simulink model "GB_and_guyan"  (R2023a)
settings: Solver=ode4  StartTime=0.0  StopTime=tend  FixedStep=dt  RelTol=1e-3
undefined symbols (not defined in the file): a0, a1, a2, a3, a4, a5, a6, a7, Ag, AgN, alpha1, alpha2, C_phys_5dof, CNrt, CRrt, delay, dt, dv1, dv2, EQ_intensity, EQ_sw, F, FN, K_phys_5dof, Kbar_inv, KNbar_inv, Koo, Kot, l, lN, M_phys_5dof, MNrt, MRrt, Muu, Phi_u, Rbar, RNbar
libraries: simulink x1, sldrtlib x1
settings Model: Creator=icu327  LastModifiedBy=liangyu
settings SolverCC: AlgebraicLoopSolver=TrustRegion
settings DataIOCC: SaveFormat=Array  ReturnWorkspaceOutputs=off
settings DebuggingCC: UnconnectedInputMsg=warning  UnconnectedOutputMsg=warning  UnconnectedLineMsg=warning  ArithmeticOperatorsInVariantConditions=warning
settings HardwareCC: ProdBitPerLong=64  ProdHWDeviceType=Intel->x86-64 (Linux 64)
settings ModelReferenceCC: EnableRefExpFcnMdlSchedulingChecks=on
settings SFSimCC: CustomCodeUndefinedFunction=UseInterfaceOnly
settings RTWCC: Description=Simulink Desktop Real-Time  SystemTargetFile=sldrt.tlc  TemplateMakefile=sldrt.tmf  RTWCompilerOptimization=on
settings CodeAppCC: MaxIdLength=95  StateflowObjectComments=on
settings SimulinkDesktopRealTimeCC: TargetLibSuffix=_sldrt.a  TargetPreCompLibLocation=C:\Program Files\MATLAB\R2023a\toolbox\sldrt\lib\win64

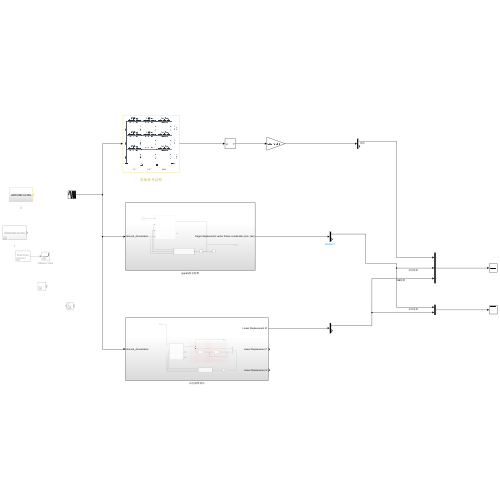
[thumbnail: Simulink's stored preview of the top-level diagram]
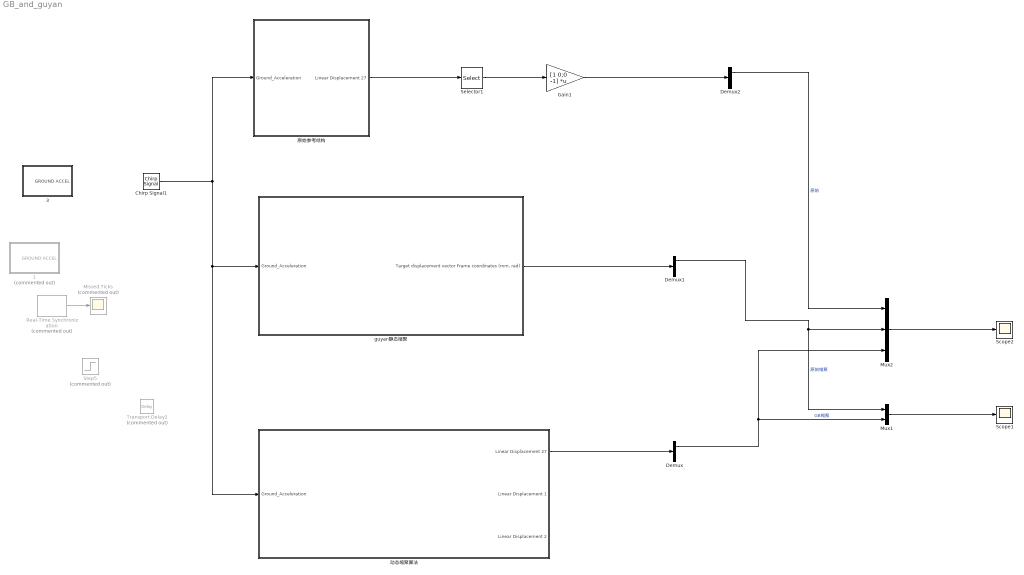
== system GB_and_guyan ==
  " 1" : Subsystem  Commented=on
  " 3" : Subsystem
  " 原始参考结构" : Subsystem
      mask Display: image('$imagefile'); % Use "Edit Image" on toolstrip to change.
  Chirp Signal1 : simulink/Sources/Chirp Signal  f1=0.1  T=60  f2=25
  Demux : Demux  Outputs=2
  Demux1 : Demux  Outputs=2
  Demux2 : Demux  Outputs=2
  Gain1 : Gain  Gain=[1 0;0 -1]  Multiplication=Matrix(K*u) (u vector)
  Missed Ticks : Scope  Commented=on
  Mux1 : Mux  Inputs=2
  Mux2 : Mux  Inputs=3
  Real-Time Synchronization : sldrtlib/Real-Time Synchronization  Commented=on  SampleTime=dt  MaxMissedTicks=10000  ShowMissedTicks=on  YieldWhenWaiting=off
  Scope1 : Scope
  Scope2 : Scope
  Selector1 : Selector  InputPortWidth=29  IndexOptions=Index vector (dialog)  Indices=[27 21]  OutputSizes=1
  Step5 : Step  Commented=on  SampleTime=0
  Transport Delay2 : TransportDelay  Commented=on  DelayTime=0.03
  guyan静态缩聚 : Subsystem
  动态缩聚算法 : Subsystem
  wires:
  Real-Time Synchronization/1 -> Missed Ticks/1
  " 原始参考结构"/1(Linear Displacement 27) -> Selector1/1
  Selector1/1 -> Gain1/1
  Chirp Signal1/1 -> 动态缩聚算法/1(Ground_Acceleration), guyan静态缩聚/1(Ground_Acceleration), " 原始参考结构"/1(Ground_Acceleration)
  Demux1/1 -> Mux2/2, Mux1/1  "原始缩聚"
  Mux1/1 -> Scope1/1
  Demux/1 -> Mux2/3, Mux1/2  "GB缩聚"
  Gain1/1 -> Demux2/1
  Demux2/1 -> Mux2/1  "原始"
  Mux2/1 -> Scope2/1
  guyan静态缩聚/1("Target displacement vector Frame coordinates (mm, rad)") -> Demux1/1
  动态缩聚算法/1(Linear Displacement 27) -> Demux/1

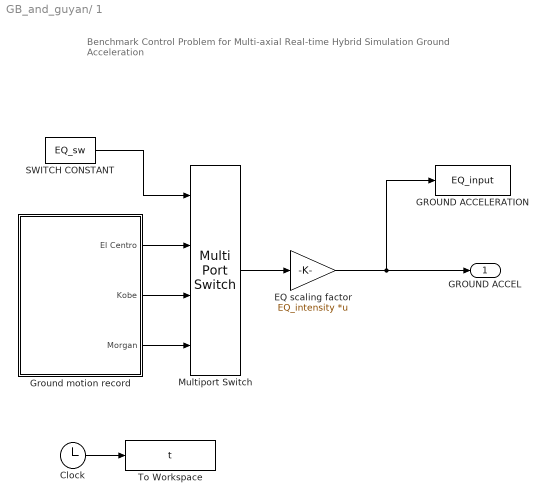
== system GB_and_guyan/ 1 ==
  note: Benchmark Control Problem for
      | Multi-axial Real-time Hybrid Simulation
      | Ground Acceleration
  Clock : Clock
  EQ scaling factor : Gain  Gain=EQ_intensity  Multiplication=Matrix(K*u)
  GROUND ACCELERATION : ToWorkspace  VariableName=EQ_input  SampleTime=-1
      settings: Save2DSignal=2-D array (concatenate along first dimension)
  Ground motion record : Subsystem
  Multiport Switch : MultiPortSwitch  SaturateOnIntegerOverflow=off  InputSameDT=off
  SWITCH CONSTANT : Constant  Value=EQ_sw
  To Workspace : ToWorkspace  VariableName=t  SampleTime=dt
  GROUND ACCEL : Outport  VectorParamsAs1DForOutWhenUnconnected=off
  wires:
  Multiport Switch/1 -> EQ scaling factor/1
  EQ scaling factor/1 -> GROUND ACCELERATION/1, GROUND ACCEL/1
  Ground motion record/1(El Centro) -> Multiport Switch/2
  Ground motion record/2(Kobe) -> Multiport Switch/3
  Ground motion record/3(Morgan) -> Multiport Switch/4
  SWITCH CONSTANT/1 -> Multiport Switch/1
  Clock/1 -> To Workspace/1

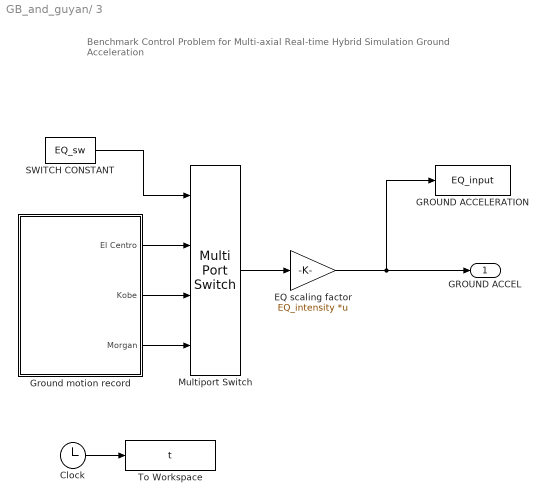
== system GB_and_guyan/ 3 ==
  note: Benchmark Control Problem for
      | Multi-axial Real-time Hybrid Simulation
      | Ground Acceleration
  Clock : Clock
  EQ scaling factor : Gain  Gain=EQ_intensity  Multiplication=Matrix(K*u)
  GROUND ACCELERATION : ToWorkspace  VariableName=EQ_input  SampleTime=-1
      settings: Save2DSignal=2-D array (concatenate along first dimension)
  Ground motion record : Subsystem
  Multiport Switch : MultiPortSwitch  SaturateOnIntegerOverflow=off  InputSameDT=off
  SWITCH CONSTANT : Constant  Value=EQ_sw
  To Workspace : ToWorkspace  VariableName=t  SampleTime=dt
  GROUND ACCEL : Outport  VectorParamsAs1DForOutWhenUnconnected=off
  wires:
  Multiport Switch/1 -> EQ scaling factor/1
  EQ scaling factor/1 -> GROUND ACCELERATION/1, GROUND ACCEL/1
  Ground motion record/1(El Centro) -> Multiport Switch/2
  Ground motion record/2(Kobe) -> Multiport Switch/3
  Ground motion record/3(Morgan) -> Multiport Switch/4
  SWITCH CONSTANT/1 -> Multiport Switch/1
  Clock/1 -> To Workspace/1

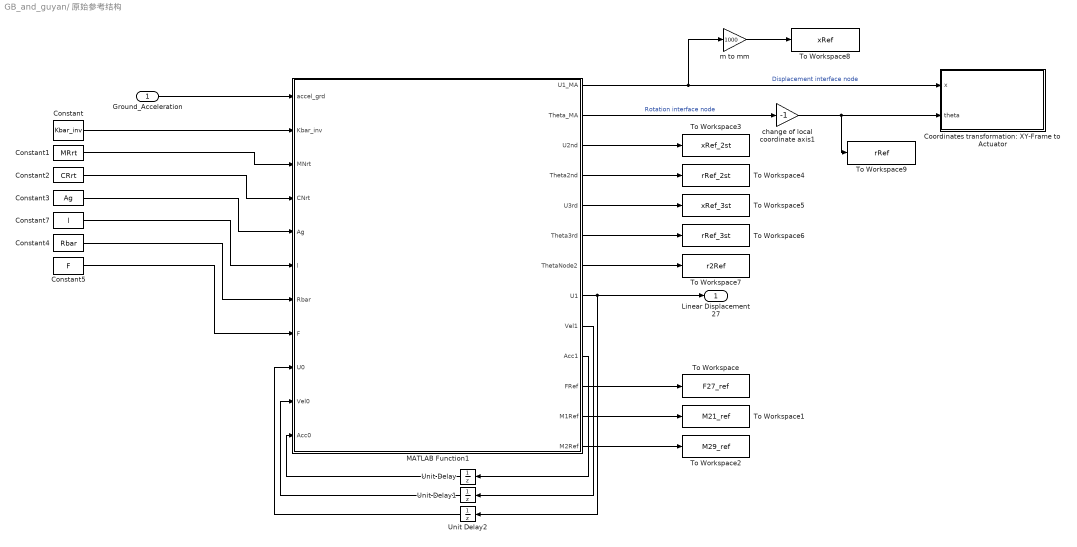
== system GB_and_guyan/ 原始参考结构 ==
  Ground_Acceleration : Inport
  Constant : Constant  Value=Kbar_inv  VectorParams1D=off
  Constant1 : Constant  Value=MRrt  VectorParams1D=off
  Constant2 : Constant  Value=CRrt  VectorParams1D=off
  Constant3 : Constant  Value=Ag  VectorParams1D=off
  Constant4 : Constant  Value=Rbar  VectorParams1D=off
  Constant5 : Constant  Value=F  VectorParams1D=off
  Constant7 : Constant  Value=l  VectorParams1D=off
  "Coordinates transformation: XY-Frame to Actuator " : Subsystem
  MATLAB Function1 : MATLAB Function  TreatAsAtomicUnit=on
  To Workspace : ToWorkspace  VariableName=F27_ref  SampleTime=-1
  To Workspace1 : ToWorkspace  VariableName=M21_ref  SampleTime=-1
  To Workspace2 : ToWorkspace  VariableName=M29_ref  SampleTime=-1
  To Workspace3 : ToWorkspace  VariableName=xRef_2st  SampleTime=dt
  To Workspace4 : ToWorkspace  VariableName=rRef_2st  SampleTime=dt
  To Workspace5 : ToWorkspace  VariableName=xRef_3st  SampleTime=dt
  To Workspace6 : ToWorkspace  VariableName=rRef_3st  SampleTime=dt
  To Workspace7 : ToWorkspace  VariableName=r2Ref  SampleTime=dt
  To Workspace8 : ToWorkspace  VariableName=xRef  SampleTime=dt
  To Workspace9 : ToWorkspace  VariableName=rRef  SampleTime=dt
  Unit Delay : UnitDelay  SampleTime=-1  HasFrameUpgradeWarning=on
  Unit Delay1 : UnitDelay  SampleTime=-1  HasFrameUpgradeWarning=on
  Unit Delay2 : UnitDelay  SampleTime=-1  HasFrameUpgradeWarning=on
  change of local coordinate axis1 : Gain  Gain=-1
  "m to mm  " : Gain  Gain=1000
  Linear Displacement 27 : Outport  VectorParamsAs1DForOutWhenUnconnected=off
  wires:
  Ground_Acceleration/1 -> MATLAB Function1/1(accel_grd)
  MATLAB Function1/1(U1_MA) -> "Coordinates transformation: XY-Frame to Actuator "/1(x), "m to mm  "/1  "Displacement interface node"
  MATLAB Function1/2(Theta_MA) -> change of local coordinate axis1/1  "Rotation interface node"
  Constant/1 -> MATLAB Function1/2(Kbar_inv)
  Constant1/1 -> MATLAB Function1/3(MNrt)
  Constant2/1 -> MATLAB Function1/4(CNrt)
  Constant3/1 -> MATLAB Function1/5(Ag)
  Constant7/1 -> MATLAB Function1/6(l)
  Constant4/1 -> MATLAB Function1/7(Rbar)
  Unit Delay2/1 -> MATLAB Function1/9(U0)
  Unit Delay1/1 -> MATLAB Function1/10(Vel0)
  Unit Delay/1 -> MATLAB Function1/11(Acc0)
  MATLAB Function1/9(Vel1) -> Unit Delay1/1
  MATLAB Function1/10(Acc1) -> Unit Delay/1
  MATLAB Function1/8(U1) -> Linear Displacement 27/1, Unit Delay2/1
  Constant5/1 -> MATLAB Function1/8(F)
  MATLAB Function1/13(M2Ref) -> To Workspace2/1
  MATLAB Function1/12(M1Ref) -> To Workspace1/1
  MATLAB Function1/11(FRef) -> To Workspace/1
  MATLAB Function1/3(U2nd) -> To Workspace3/1
  MATLAB Function1/4(Theta2nd) -> To Workspace4/1
  MATLAB Function1/5(U3rd) -> To Workspace5/1
  MATLAB Function1/6(Theta3rd) -> To Workspace6/1
  MATLAB Function1/7(ThetaNode2) -> To Workspace7/1
  "m to mm  "/1 -> To Workspace8/1
  change of local coordinate axis1/1 -> To Workspace9/1, "Coordinates transformation: XY-Frame to Actuator "/2(theta)

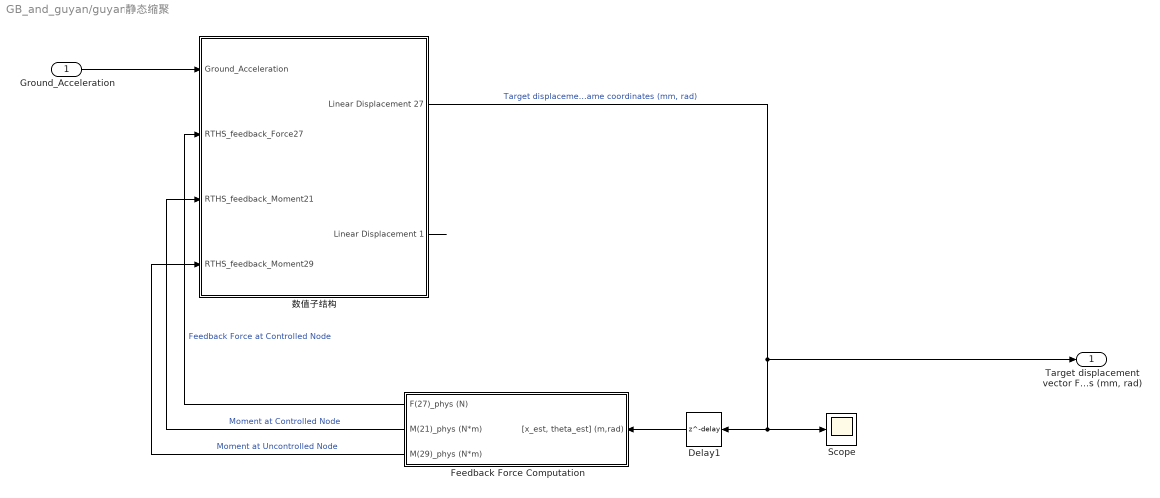
== system GB_and_guyan/guyan静态缩聚 ==
  Ground_Acceleration : Inport
  " 数值子结构" : Subsystem
      mask Display: image('$imagefile'); % Use "Edit Image" on toolstrip to change.
  Delay1 : Delay  DelayLength=delay
  Feedback Force Computation : Subsystem
  Scope : Scope
  "Target displacement vector Frame coordinates (mm, rad)" : Outport
  wires:
  Feedback Force Computation/2(M(21)_phys (N*m)) -> " 数值子结构"/3(RTHS_feedback_Moment21)  "Moment at Controlled Node"
  " 数值子结构"/1(Linear Displacement 27) -> "Target displacement vector Frame coordinates (mm, rad)"/1, Scope/1, Delay1/1  "Target displacement vector Frame coordinates (mm, rad)"
  Ground_Acceleration/1 -> " 数值子结构"/1(Ground_Acceleration)
  Feedback Force Computation/1(F(27)_phys (N)) -> " 数值子结构"/2(RTHS_feedback_Force27)  "Feedback Force at Controlled Node"
  Delay1/1 -> Feedback Force Computation/1("[x_est, theta_est] (m,rad)")
  Feedback Force Computation/3(M(29)_phys (N*m)) -> " 数值子结构"/4(RTHS_feedback_Moment29)  "Moment at Uncontrolled Node"
  " 数值子结构"/2(Linear Displacement 1) -> ?

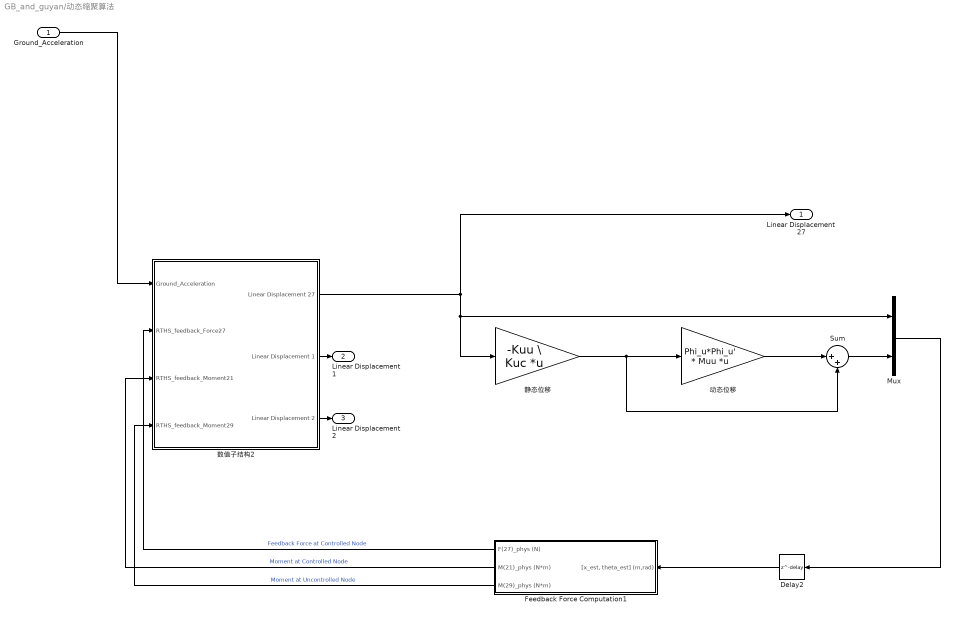
== system GB_and_guyan/动态缩聚算法 ==
  Ground_Acceleration : Inport
  " 数值子结构2" : Subsystem
      mask Display: image('$imagefile'); % Use "Edit Image" on toolstrip to change.
  Delay2 : Delay  DelayLength=delay
  Feedback Force Computation1 : Subsystem
  Mux : Mux  Inputs=2
  Sum : Sum  Inputs=|++
  动态位移 : Gain  Gain=Phi_u*Phi_u' * Muu  Multiplication=Matrix(K*u) (u vector)
  静态位移 : Gain  Gain=-Kuu \ Kuc  Multiplication=Matrix(K*u) (u vector)
  Linear Displacement 27 : Outport
  Linear Displacement 1 : Outport  Port=2
  Linear Displacement 2 : Outport  Port=3
  wires:
  动态位移/1 -> Sum/1
  " 数值子结构2"/1(Linear Displacement 27) -> Linear Displacement 27/1, 静态位移/1, Mux/1
  Feedback Force Computation1/3(M(29)_phys (N*m)) -> " 数值子结构2"/4(RTHS_feedback_Moment29)  "Moment at Uncontrolled Node"
  Mux/1 -> Delay2/1
  静态位移/1 -> 动态位移/1, Sum/2
  Sum/1 -> Mux/2
  Feedback Force Computation1/2(M(21)_phys (N*m)) -> " 数值子结构2"/3(RTHS_feedback_Moment21)  "Moment at Controlled Node"
  Delay2/1 -> Feedback Force Computation1/1("[x_est, theta_est] (m,rad)")
  Feedback Force Computation1/1(F(27)_phys (N)) -> " 数值子结构2"/2(RTHS_feedback_Force27)  "Feedback Force at Controlled Node"
  " 数值子结构2"/2(Linear Displacement 1) -> Linear Displacement 1/1
  " 数值子结构2"/3(Linear Displacement 2) -> Linear Displacement 2/1
  Ground_Acceleration/1 -> " 数值子结构2"/1(Ground_Acceleration)

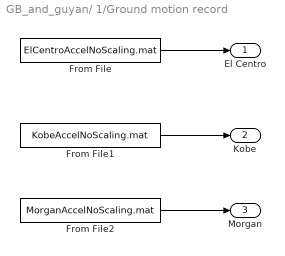
== system GB_and_guyan/ 1/Ground motion record ==
  From File : FromFile  FileName=ElCentroAccelNoScaling.mat  SampleTime=dt
  From File1 : FromFile  FileName=KobeAccelNoScaling.mat  SampleTime=dt
  From File2 : FromFile  FileName=MorganAccelNoScaling.mat  SampleTime=dt
  El Centro : Outport
  Kobe : Outport  Port=2
  Morgan : Outport  Port=3
  wires:
  From File/1 -> El Centro/1
  From File2/1 -> Morgan/1
  From File1/1 -> Kobe/1

== system GB_and_guyan/ 3/Ground motion record ==
  From File : FromFile  FileName=D:\matlab\LY\gitee\liangyustability\simulink模型修改\Ground_motions\ElCentroAccelNoScaling.mat  SampleTime=dt
  From File1 : FromFile  FileName=D:\matlab\LY\gitee\liangyustability\simulink模型修改\Ground_motions\KobeAccelNoScaling.mat  SampleTime=dt
  From File2 : FromFile  FileName=D:\matlab\LY\gitee\liangyustability\simulink模型修改\Ground_motions\MorganAccelNoScaling.mat  SampleTime=dt
  El Centro : Outport
  Kobe : Outport  Port=2
  Morgan : Outport  Port=3
  wires:
  From File/1 -> El Centro/1
  From File2/1 -> Morgan/1
  From File1/1 -> Kobe/1

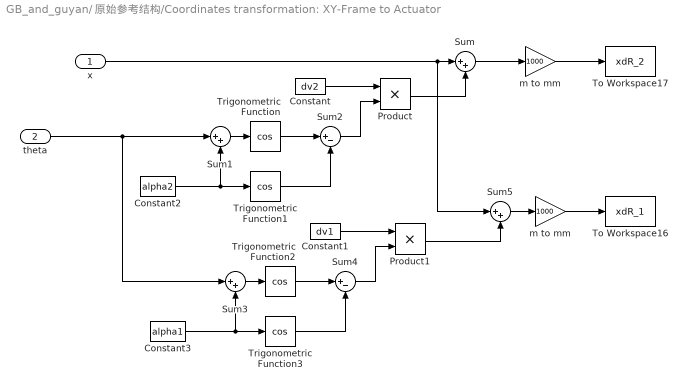
== system GB_and_guyan/ 原始参考结构/Coordinates transformation: XY-Frame to Actuator  ==
  x : Inport
  theta : Inport  Port=2
  Constant : Constant  Value=dv2
  Constant1 : Constant  Value=dv1
  Constant2 : Constant  Value=alpha2
  Constant3 : Constant  Value=alpha1
  Product : Product
  Product1 : Product
  Sum{,1,3,5} (4 alike) : Sum  Inputs=|++
  Sum2 : Sum  Inputs=|+-
  Sum4 : Sum  Inputs=|+-
  To Workspace16 : ToWorkspace  VariableName=xdR_1  SampleTime=dt
  To Workspace17 : ToWorkspace  VariableName=xdR_2  SampleTime=dt
  Trigonometric Function{,1..3} (4 alike) : Trigonometry  Operator=cos
  m to mm : Gain  Gain=1000
  "m to mm " : Gain  Gain=1000
  wires:
  theta/1 -> Sum1/1, Sum3/1
  "m to mm "/1 -> To Workspace16/1
  m to mm/1 -> To Workspace17/1
  Sum5/1 -> "m to mm "/1
  Product1/1 -> Sum5/2
  Constant1/1 -> Product1/1
  Constant3/1 -> Trigonometric Function3/1, Sum3/2
  Sum3/1 -> Trigonometric Function2/1
  Trigonometric Function2/1 -> Sum4/1
  Trigonometric Function3/1 -> Sum4/2
  Sum4/1 -> Product1/2
  Sum/1 -> m to mm/1
  Product/1 -> Sum/2
  Sum2/1 -> Product/2
  Trigonometric Function1/1 -> Sum2/2
  Trigonometric Function/1 -> Sum2/1
  Sum1/1 -> Trigonometric Function/1
  Constant2/1 -> Trigonometric Function1/1, Sum1/2
  Constant/1 -> Product/1
  x/1 -> Sum/1, Sum5/1

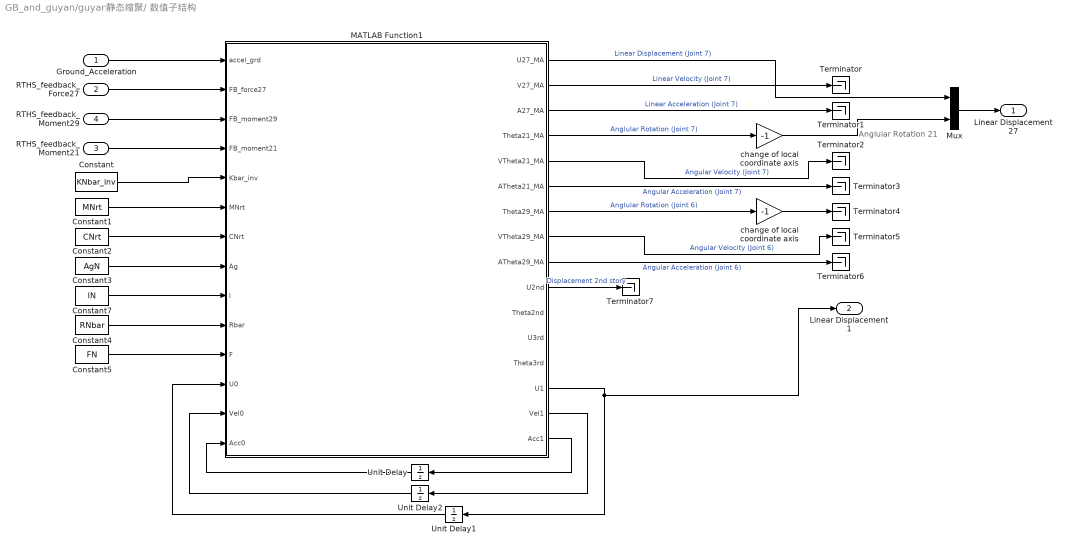
== system GB_and_guyan/guyan静态缩聚/ 数值子结构 ==
  note: Anglular Rotation 21
  Ground_Acceleration : Inport
  RTHS_feedback_Force27 : Inport  Port=2
  RTHS_feedback_Moment21 : Inport  Port=3
  RTHS_feedback_Moment29 : Inport  Port=4
  Constant : Constant  Value=KNbar_inv  VectorParams1D=off
  Constant1 : Constant  Value=MNrt  VectorParams1D=off
  Constant2 : Constant  Value=CNrt  VectorParams1D=off
  Constant3 : Constant  Value=AgN  VectorParams1D=off
  Constant4 : Constant  Value=RNbar  VectorParams1D=off
  Constant5 : Constant  Value=FN  VectorParams1D=off
  Constant7 : Constant  Value=lN  VectorParams1D=off
  MATLAB Function1 : MATLAB Function  TreatAsAtomicUnit=on
  Mux : Mux  Inputs=2
  Terminator{,1..7} (8 alike) : Terminator
  Unit Delay : UnitDelay  SampleTime=-1  HasFrameUpgradeWarning=on
  Unit Delay1 : UnitDelay  SampleTime=-1  HasFrameUpgradeWarning=on
  Unit Delay2 : UnitDelay  SampleTime=-1  HasFrameUpgradeWarning=on
  change of local coordinate axis : Gain  Gain=-1
  "change of local coordinate axis  " : Gain  Gain=-1
  Linear Displacement 27 : Outport  VectorParamsAs1DForOutWhenUnconnected=off
  Linear Displacement 1 : Outport  Port=2  VectorParamsAs1DForOutWhenUnconnected=off
  wires:
  Ground_Acceleration/1 -> MATLAB Function1/1(accel_grd)
  RTHS_feedback_Force27/1 -> MATLAB Function1/2(FB_force27)
  RTHS_feedback_Moment29/1 -> MATLAB Function1/3(FB_moment29)
  MATLAB Function1/1(U27_MA) -> Mux/1  "Linear Displacement (Joint 7)"
  MATLAB Function1/4(Theta21_MA) -> change of local coordinate axis/1  "Anglular Rotation (Joint 7)"
  Constant/1 -> MATLAB Function1/5(Kbar_inv)
  Constant1/1 -> MATLAB Function1/6(MNrt)
  Constant2/1 -> MATLAB Function1/7(CNrt)
  Constant3/1 -> MATLAB Function1/8(Ag)
  Constant7/1 -> MATLAB Function1/9(l)
  Constant4/1 -> MATLAB Function1/10(Rbar)
  Unit Delay1/1 -> MATLAB Function1/12(U0)
  Unit Delay2/1 -> MATLAB Function1/13(Vel0)
  Unit Delay/1 -> MATLAB Function1/14(Acc0)
  MATLAB Function1/15(Vel1) -> Unit Delay2/1
  MATLAB Function1/16(Acc1) -> Unit Delay/1
  Constant5/1 -> MATLAB Function1/11(F)
  MATLAB Function1/2(V27_MA) -> Terminator/1  "Linear Velocity (Joint 7)"
  MATLAB Function1/3(A27_MA) -> Terminator1/1  "Linear Acceleration (Joint 7)"
  MATLAB Function1/5(VTheta21_MA) -> Terminator2/1  "Angular Velocity (Joint 7)"
  MATLAB Function1/6(ATheta21_MA) -> Terminator3/1  "Angular Acceleration (Joint 7)"
  MATLAB Function1/9(ATheta29_MA) -> Terminator6/1  "Angular Acceleration (Joint 6)"
  MATLAB Function1/8(VTheta29_MA) -> Terminator5/1  "Angular Velocity (Joint 6)"
  MATLAB Function1/7(Theta29_MA) -> "change of local coordinate axis  "/1  "Anglular Rotation (Joint 6)"
  RTHS_feedback_Moment21/1 -> MATLAB Function1/4(FB_moment21)
  change of local coordinate axis/1 -> Mux/2
  "change of local coordinate axis  "/1 -> Terminator4/1
  Mux/1 -> Linear Displacement 27/1
  MATLAB Function1/10(U2nd) -> Terminator7/1  "Displacement 2nd story"
  MATLAB Function1/14(U1) -> Linear Displacement 1/1, Unit Delay1/1

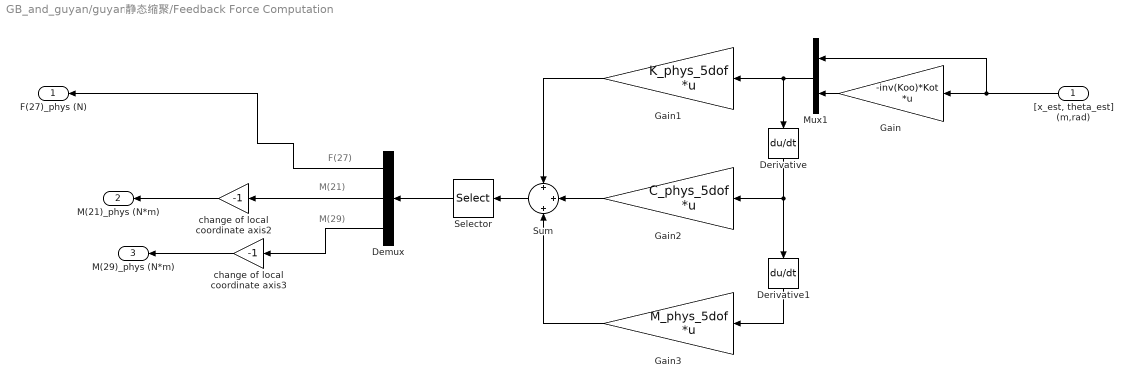
== system GB_and_guyan/guyan静态缩聚/Feedback Force Computation ==
  note: F(27)
  note: M(21)
  note: M(29)
  "[x_est, theta_est] (m,rad)" : Inport
  Demux : Demux  Outputs=3
  Derivative : Derivative
  Derivative1 : Derivative
  Gain : Gain  Gain=-inv(Koo)*Kot  Multiplication=Matrix(K*u) (u vector)
  Gain1 : Gain  Gain=K_phys_5dof  Multiplication=Matrix(K*u) (u vector)
  Gain2 : Gain  Gain=C_phys_5dof  Multiplication=Matrix(K*u) (u vector)
  Gain3 : Gain  Gain=M_phys_5dof  Multiplication=Matrix(K*u) (u vector)
  Mux1 : Mux  Inputs=2
  Selector : Selector  InputPortWidth=5  IndexOptions=Index vector (dialog)  Indices=[1 2 3]  OutputSizes=1
  Sum : Sum  Inputs=+|+|+
  change of local coordinate axis2 : Gain  Gain=-1
  change of local coordinate axis3 : Gain  Gain=-1
  F(27)_phys (N) : Outport  VectorParamsAs1DForOutWhenUnconnected=off
  M(21)_phys (N*m) : Outport  Port=2  VectorParamsAs1DForOutWhenUnconnected=off
  M(29)_phys (N*m) : Outport  Port=3  VectorParamsAs1DForOutWhenUnconnected=off
  wires:
  Gain/1 -> Mux1/2
  Derivative1/1 -> Gain3/1
  Gain2/1 -> Sum/2
  Derivative/1 -> Gain2/1, Derivative1/1
  Gain1/1 -> Sum/1
  "[x_est, theta_est] (m,rad)"/1 -> Gain/1, Mux1/1
  Demux/1 -> F(27)_phys (N)/1
  Sum/1 -> Selector/1
  Selector/1 -> Demux/1
  Gain3/1 -> Sum/3
  Demux/2 -> change of local coordinate axis2/1
  Demux/3 -> change of local coordinate axis3/1
  Mux1/1 -> Derivative/1, Gain1/1
  change of local coordinate axis2/1 -> M(21)_phys (N*m)/1
  change of local coordinate axis3/1 -> M(29)_phys (N*m)/1

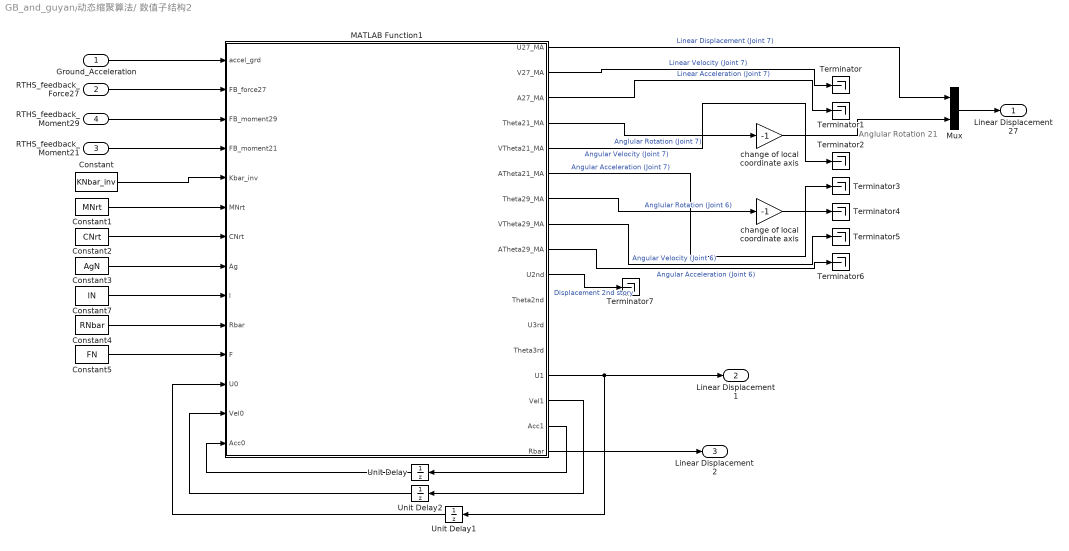
== system GB_and_guyan/动态缩聚算法/ 数值子结构2 ==
  note: Anglular Rotation 21
  Ground_Acceleration : Inport
  RTHS_feedback_Force27 : Inport  Port=2
  RTHS_feedback_Moment21 : Inport  Port=3
  RTHS_feedback_Moment29 : Inport  Port=4
  Constant : Constant  Value=KNbar_inv  VectorParams1D=off
  Constant1 : Constant  Value=MNrt  VectorParams1D=off
  Constant2 : Constant  Value=CNrt  VectorParams1D=off
  Constant3 : Constant  Value=AgN  VectorParams1D=off
  Constant4 : Constant  Value=RNbar  VectorParams1D=off
  Constant5 : Constant  Value=FN  VectorParams1D=off
  Constant7 : Constant  Value=lN  VectorParams1D=off
  MATLAB Function1 : MATLAB Function  TreatAsAtomicUnit=on
  Mux : Mux  Inputs=2
  Terminator{,1..7} (8 alike) : Terminator
  Unit Delay : UnitDelay  SampleTime=-1  HasFrameUpgradeWarning=on
  Unit Delay1 : UnitDelay  SampleTime=-1  HasFrameUpgradeWarning=on
  Unit Delay2 : UnitDelay  SampleTime=-1  HasFrameUpgradeWarning=on
  change of local coordinate axis : Gain  Gain=-1
  "change of local coordinate axis  " : Gain  Gain=-1
  Linear Displacement 27 : Outport  VectorParamsAs1DForOutWhenUnconnected=off
  Linear Displacement 1 : Outport  Port=2  VectorParamsAs1DForOutWhenUnconnected=off
  Linear Displacement 2 : Outport  Port=3  VectorParamsAs1DForOutWhenUnconnected=off
  wires:
  Ground_Acceleration/1 -> MATLAB Function1/1(accel_grd)
  RTHS_feedback_Force27/1 -> MATLAB Function1/2(FB_force27)
  RTHS_feedback_Moment29/1 -> MATLAB Function1/3(FB_moment29)
  MATLAB Function1/1(U27_MA) -> Mux/1  "Linear Displacement (Joint 7)"
  MATLAB Function1/4(Theta21_MA) -> change of local coordinate axis/1  "Anglular Rotation (Joint 7)"
  Constant/1 -> MATLAB Function1/5(Kbar_inv)
  Constant1/1 -> MATLAB Function1/6(MNrt)
  Constant2/1 -> MATLAB Function1/7(CNrt)
  Constant3/1 -> MATLAB Function1/8(Ag)
  Constant7/1 -> MATLAB Function1/9(l)
  Constant4/1 -> MATLAB Function1/10("Rbar ")
  Unit Delay1/1 -> MATLAB Function1/12(U0)
  Unit Delay2/1 -> MATLAB Function1/13(Vel0)
  Unit Delay/1 -> MATLAB Function1/14(Acc0)
  MATLAB Function1/15(Vel1) -> Unit Delay2/1
  MATLAB Function1/16(Acc1) -> Unit Delay/1
  Constant5/1 -> MATLAB Function1/11(F)
  MATLAB Function1/2(V27_MA) -> Terminator/1  "Linear Velocity (Joint 7)"
  MATLAB Function1/3(A27_MA) -> Terminator1/1  "Linear Acceleration (Joint 7)"
  MATLAB Function1/5(VTheta21_MA) -> Terminator2/1  "Angular Velocity (Joint 7)"
  MATLAB Function1/6(ATheta21_MA) -> Terminator3/1  "Angular Acceleration (Joint 7)"
  MATLAB Function1/9(ATheta29_MA) -> Terminator6/1  "Angular Acceleration (Joint 6)"
  MATLAB Function1/8(VTheta29_MA) -> Terminator5/1  "Angular Velocity (Joint 6)"
  MATLAB Function1/7(Theta29_MA) -> "change of local coordinate axis  "/1  "Anglular Rotation (Joint 6)"
  RTHS_feedback_Moment21/1 -> MATLAB Function1/4(FB_moment21)
  change of local coordinate axis/1 -> Mux/2
  "change of local coordinate axis  "/1 -> Terminator4/1
  Mux/1 -> Linear Displacement 27/1
  MATLAB Function1/10(U2nd) -> Terminator7/1  "Displacement 2nd story"
  MATLAB Function1/14(U1) -> Unit Delay1/1, Linear Displacement 1/1
  MATLAB Function1/17(Rbar) -> Linear Displacement 2/1

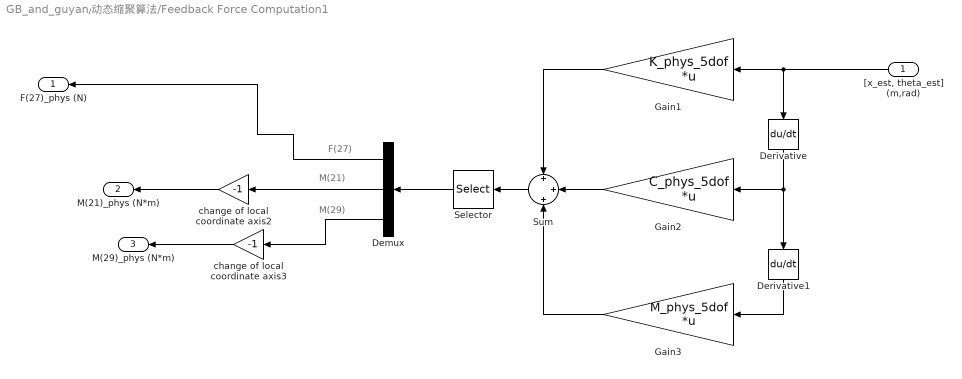
== system GB_and_guyan/动态缩聚算法/Feedback Force Computation1 ==
  note: F(27)
  note: M(21)
  note: M(29)
  "[x_est, theta_est] (m,rad)" : Inport
  Demux : Demux  Outputs=3
  Derivative : Derivative
  Derivative1 : Derivative
  Gain1 : Gain  Gain=K_phys_5dof  Multiplication=Matrix(K*u) (u vector)
  Gain2 : Gain  Gain=C_phys_5dof  Multiplication=Matrix(K*u) (u vector)
  Gain3 : Gain  Gain=M_phys_5dof  Multiplication=Matrix(K*u) (u vector)
  Selector : Selector  InputPortWidth=5  IndexOptions=Index vector (dialog)  Indices=[1 2 3]  OutputSizes=1
  Sum : Sum  Inputs=+|+|+
  change of local coordinate axis2 : Gain  Gain=-1
  change of local coordinate axis3 : Gain  Gain=-1
  F(27)_phys (N) : Outport  VectorParamsAs1DForOutWhenUnconnected=off
  M(21)_phys (N*m) : Outport  Port=2  VectorParamsAs1DForOutWhenUnconnected=off
  M(29)_phys (N*m) : Outport  Port=3  VectorParamsAs1DForOutWhenUnconnected=off
  wires:
  Derivative1/1 -> Gain3/1
  Gain2/1 -> Sum/2
  Derivative/1 -> Gain2/1, Derivative1/1
  Gain1/1 -> Sum/1
  Demux/1 -> F(27)_phys (N)/1
  Sum/1 -> Selector/1
  Selector/1 -> Demux/1
  Gain3/1 -> Sum/3
  Demux/2 -> change of local coordinate axis2/1
  Demux/3 -> change of local coordinate axis3/1
  "[x_est, theta_est] (m,rad)"/1 -> Derivative/1, Gain1/1
  change of local coordinate axis2/1 -> M(21)_phys (N*m)/1
  change of local coordinate axis3/1 -> M(29)_phys (N*m)/1

== matlab function GB_and_guyan/ 原始参考结构/MATLAB Function1 ==
  data: U1_MA output; Theta_MA output; U2nd output; Theta2nd output; U3rd output; Theta3rd output; ThetaNode2 output; U1 output; Vel1 output; Acc1 output; accel_grd input; Kbar_inv input; MNrt input; CNrt input; Ag input; l input; Rbar input; F input; U0 input; Vel0 input; Acc0 input; a0 parameter; a1 parameter; a2 parameter; a3 parameter; a4 parameter; a5 parameter; a6 parameter; a7 parameter; FRef output; M1Ref output; M2Ref output
function [U1_MA,Theta_MA,U2nd,Theta2nd,U3rd,Theta3rd,ThetaNode2, U1,Vel1,Acc1,FRef,M1Ref,M2Ref]=fcn(accel_grd,Kbar_inv, MNrt, CNrt,Ag,l,Rbar,F,...
    U0,Vel0,Acc0, a0, a1, a2, a3, a4, a5, a6, a7)
             
             
    % ============================
	% *  Update next iteration   *
	% ============================
    ndof = length(Kbar_inv);
    U1   = zeros(ndof,1);
    Vel1 = zeros(ndof,1);
    Acc1 = zeros(ndof,1);
    U1_MA = 0;
    Theta_MA = 0;
    FRef = 0;
    M1Ref = 0;
    M2Ref = 0;

     U2nd= 0;
    Theta2nd= 0;
    U3rd=0;
    Theta3rd=0;
    ThetaNode2=0;
    
    % ============================
	% *  Feedback Force / Moment *
	% ============================
%     F(27) = -FB_force;
%     F(14) = -FB_moment;

    % ==========================
	% *     Update Matrices    *
	% ==========================
    Ag(:)  = accel_grd * l;
    
   	% ==========================
	% * 	  Form Rbar  	   *
	% ==========================
	Rbar = ( (MNrt * ((a0*U0)+(a2*Vel0)+(a3*Acc0))) + ...
		     (CNrt * ((a1*U0)+(a4*Vel0)+(a5*Acc0))) - F - (MNrt * Ag) );
    FRef = Rbar(27);
    M1Ref= Rbar(21);
    M2Ref= Rbar(29);
    % ==========================
	% * Solve for Displacement *
	% ==========================
	U1 = Kbar_inv * Rbar;
    
	% ============================
	% * Compute Velocity & Accel *
	% ============================
	Acc1=a0*(U1-U0)-a2*Vel0-a3*Acc0;
	Vel1=Vel0+a7*Acc1+a6*Acc0; 

	% ============================
	% *    Output u1 and theta   *
	% ============================
    U1_MA    = U1(27);
    Theta_MA = U1(21);

    % ============================
	% *  Upper Stories Response  *
	% ============================
    U2nd = U1(26);              %Displacement 2nd story, node 12, DOF 26
    Theta2nd = U1(22);          %Rotation 2nd story, node 12, DOF 22
    U3rd = U1(13);              %Displacement 3rd story, node 16, DOF 13
    Theta3rd = U1(3);           %Rotation 3rd story, node 16, DOF 3
    ThetaNode2 = U1(29);        %Rotation 2nd node of the common interface, node 6, DOF 29

end

== matlab function GB_and_guyan/guyan静态缩聚/ 数值子结构/MATLAB Function1 ==
  data: U27_MA output; V27_MA output; A27_MA output; Theta21_MA output; VTheta21_MA output; ATheta21_MA output; Theta29_MA output; VTheta29_MA output; ATheta29_MA output; U2nd output; Theta2nd output; U3rd output; Theta3rd output; U1 output; Vel1 output; Acc1 output; accel_grd input; FB_force27 input; FB_moment29 input; FB_moment21 input; Kbar_inv input; MNrt input; CNrt input; Ag input; l input; Rbar input; F input; U0 input; Vel0 input; Acc0 input; a0 parameter; a1 parameter; a2 parameter; a3 parameter; a4 parameter; a5 parameter; a6 parameter; a7 parameter
function [U27_MA,V27_MA,A27_MA,Theta21_MA,VTheta21_MA,ATheta21_MA,Theta29_MA,VTheta29_MA,ATheta29_MA,U2nd,Theta2nd,U3rd,Theta3rd,U1,Vel1,Acc1]=...
    fcn(accel_grd,FB_force27,FB_moment29,FB_moment21,Kbar_inv, MNrt, CNrt,Ag,l,Rbar,F,...
    U0,Vel0,Acc0, a0, a1, a2, a3, a4, a5, a6, a7)
             
             
    % ============================
	% *  Update next iteration   *
	% ============================
    ndof = length(Kbar_inv);
    U1   = zeros(ndof,1);
    Vel1 = zeros(ndof,1);
    Acc1 = zeros(ndof,1);
    
    U27_MA = 0;
    V27_MA = 0;
    A27_MA = 0;

    Theta21_MA = 0;
    VTheta21_MA = 0;
    ATheta21_MA = 0;
% 
%     U6_MA = 0;
%     V6_MA = 0;
%     A6_MA = 0;
    U2nd = 0 ;              %Displacement 2nd story, node 12, DOF 26
    Theta2nd = 0;          %Rotation 2nd story, node 12, DOF 22
    U3rd = 0;              %Displacement 3rd story, node 16, DOF 13
    Theta3rd = 0;           %Rotation 3rd story, node 16, DOF 3


    Theta29_MA = 0;
    VTheta29_MA = 0;
    ATheta29_MA = 0;

    % ============================
	% *  Feedback Force / Moment *
	% ============================
    F(27) = FB_force27;
    F(21) = FB_moment21;
    F(29) = FB_moment29;

    % ==========================
	% *     Update Matrices    *
	% ==========================
    Ag(:)  = accel_grd * l;
    
   	% ==========================
	% * 	  Form Rbar  	   *
	% ==========================
	Rbar = ( (MNrt * ((a0*U0)+(a2*Vel0)+(a3*Acc0))) + ...
		     (CNrt * ((a1*U0)+(a4*Vel0)+(a5*Acc0))) - F - (MNrt * Ag) );
    
    % ==========================
	% * Solve for Displacement *
	% ==========================
	U1 = Kbar_inv * Rbar;
    
	% ============================
	% * Compute Velocity & Accel *
	% ============================
	Acc1=a0*(U1-U0)-a2*Vel0-a3*Acc0;
	Vel1=Vel0+a7*Acc1+a6*Acc0; 

	% ============================
	% *    Output u1 and theta   *
	% ============================
    U27_MA    = U1(27);
    V27_MA    = Vel1(27);
    A27_MA    = Acc1(27);    

%     U6_MA    = U1(27);
%     V6_MA    = Vel1(27);
%     A6_MA    = Acc1(27);

    Theta21_MA = U1(21);
    VTheta21_MA = Vel1(21);
    ATheta21_MA = Acc1(21);

    Theta29_MA = U1(29);
    VTheta29_MA = Vel1(29);
    ATheta29_MA = Acc1(29);
    
    % ADDED by Johnny
    U2nd = U1(26);              %Displacement 2nd story, node 12, DOF 26
    Theta2nd = U1(22);          %Rotation 2nd story, node 12, DOF 22
    U3rd = U1(13);              %Displacement 3rd story, node 16, DOF 13
    Theta3rd = U1(3);           %Rotation 3rd story, node 16, DOF 3

end

== matlab function GB_and_guyan/动态缩聚算法/ 数值子结构2/MATLAB Function1 ==
  data: U27_MA output; V27_MA output; A27_MA output; Theta21_MA output; VTheta21_MA output; ATheta21_MA output; Theta29_MA output; VTheta29_MA output; ATheta29_MA output; U2nd output; Theta2nd output; U3rd output; Theta3rd output; U1 output; Vel1 output; Acc1 output; accel_grd input; FB_force27 input; FB_moment29 input; FB_moment21 input; Kbar_inv input; MNrt input; CNrt input; Ag input; l input; Rbar input; F input; U0 input; Vel0 input; Acc0 input; a0 parameter; a1 parameter; a2 parameter; a3 parameter; a4 parameter; a5 parameter; a6 parameter; a7 parameter; Rbar output
function [U27_MA,V27_MA,A27_MA,Theta21_MA,VTheta21_MA,ATheta21_MA,Theta29_MA,VTheta29_MA,ATheta29_MA,U2nd,Theta2nd,U3rd,Theta3rd,U1,Vel1,Acc1,Rbar]=...
    fcn(accel_grd,FB_force27,FB_moment29,FB_moment21,Kbar_inv, MNrt, CNrt,Ag,l,Rbar,F,...
    U0,Vel0,Acc0, a0, a1, a2, a3, a4, a5, a6, a7)
             
             
    % ============================
	% *  Update next iteration   *
	% ============================
    ndof = length(Kbar_inv);
    U1   = zeros(ndof,1);
    Vel1 = zeros(ndof,1);
    Acc1 = zeros(ndof,1);
    
    U27_MA = 0;
    V27_MA = 0;
    A27_MA = 0;

    Theta21_MA = 0;
    VTheta21_MA = 0;
    ATheta21_MA = 0;
% 
%     U6_MA = 0;
%     V6_MA = 0;
%     A6_MA = 0;
    U2nd = 0 ;              %Displacement 2nd story, node 12, DOF 26
    Theta2nd = 0;          %Rotation 2nd story, node 12, DOF 22
    U3rd = 0;              %Displacement 3rd story, node 16, DOF 13
    Theta3rd = 0;           %Rotation 3rd story, node 16, DOF 3


    Theta29_MA = 0;
    VTheta29_MA = 0;
    ATheta29_MA = 0;

    % ============================
	% *  Feedback Force / Moment *
	% ============================
    F(27) = FB_force27;
    F(21) = FB_moment21;
    F(29) = FB_moment29;

    % ==========================
	% *     Update Matrices    *
	% ==========================
    Ag(:)  = accel_grd * l;
    
   	% ==========================
	% * 	  Form Rbar  	   *
	% ==========================
	Rbar = ( (MNrt * ((a0*U0)+(a2*Vel0)+(a3*Acc0))) + ...
		     (CNrt * ((a1*U0)+(a4*Vel0)+(a5*Acc0))) - F - (MNrt * Ag) );
    
    % ==========================
	% * Solve for Displacement *
	% ==========================
	U1 = Kbar_inv * Rbar;
    
	% ============================
	% * Compute Velocity & Accel *
	% ============================
	Acc1=a0*(U1-U0)-a2*Vel0-a3*Acc0;
	Vel1=Vel0+a7*Acc1+a6*Acc0; 

	% ============================
	% *    Output u1 and theta   *
	% ============================
    U27_MA    = U1(27);
    V27_MA    = Vel1(27);
    A27_MA    = Acc1(27);    

%     U6_MA    = U1(27);
%     V6_MA    = Vel1(27);
%     A6_MA    = Acc1(27);

    Theta21_MA = U1(21);
    VTheta21_MA = Vel1(21);
    ATheta21_MA = Acc1(21);

    Theta29_MA = U1(29);
    VTheta29_MA = Vel1(29);
    ATheta29_MA = Acc1(29);
    
    % ADDED by Johnny
    U2nd = U1(26);              %Displacement 2nd story, node 12, DOF 26
    Theta2nd = U1(22);          %Rotation 2nd story, node 12, DOF 22
    U3rd = U1(13);              %Displacement 3rd story, node 16, DOF 13
    Theta3rd = U1(3);           %Rotation 3rd story, node 16, DOF 3

end
